simulink model "Cw3"  (R2016b)
settings: Solver=VariableStepDiscrete  StartTime=0.0  StopTime=160e-6  RelTol=1e-3
libraries: commseqgen3 x3, dspsrcs4 x2, simulink x1, commfilt2 x1, commutil2 x1
settings Model: Creator=Krzysztof  LastModifiedBy=Krzysztof

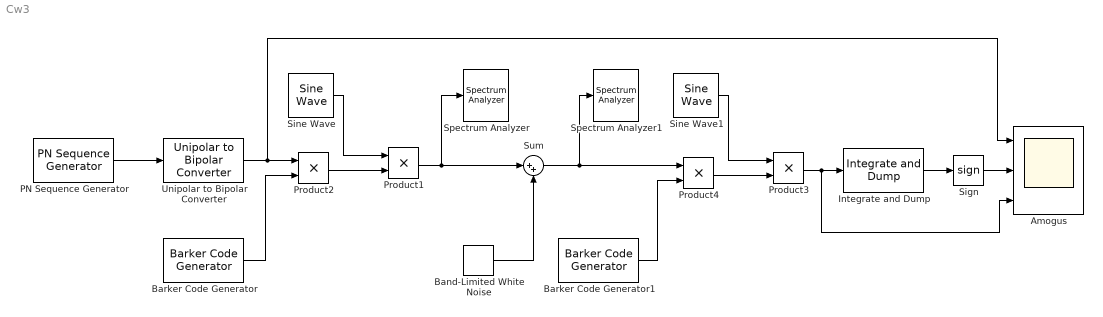
== system Cw3 ==
  "Amogus " : Scope  NumInputPorts=3
  Band-Limited White Noise : simulink/Sources/Band-Limited White Noise  Cov=[1e-11]  Ts=0.1e-9  seed=[23341]
  Barker Code Generator : commseqgen3/Barker Code Generator  Length=7  LengthSimulink=11  SampleTime=1/11e6  SamplesPerFrame=1  OutputDataType=double  SimulateUsing=Code generation
  Barker Code Generator1 : commseqgen3/Barker Code Generator  Length=7  LengthSimulink=7  SampleTime=1/11e6  SamplesPerFrame=1  OutputDataType=double  SimulateUsing=Code generation
  Integrate and Dump : commfilt2/Integrate and Dump  obssamples=10000  offsetsamples=0  nodump=off  roundingMode=Floor  overflowMode=off  outputDataTypeStr=Inherit: Same as accumulator  outputLastDataTypeStr=Inherit: Same as accumulator
  PN Sequence Generator : commseqgen3/PN Sequence Generator  poly='z^6 + z + 1'  ini_sta=[0 0 0 0 0 1]  outBitMaskSource=Dialog parameter  shift=0  outVarSiz=off  maxOutSizeMode=Dialog parameter  maxOutSize=[10 1]  Ts=1/1e6  sampPerFrame=1  reset=off  bitPackedOutputs=off  outDataType=double  numPackedBits=8  bitPackDataSigned=off  bitPackedOutDType=double
  Product1 : Product  SampleTime=0.1e-9
  Product2 : Product  SampleTime=1/11e6
  Product3 : Product  SampleTime=0.1e-9
  Product4 : Product  SampleTime=0.1e-9
  Sign : Signum
  Sine Wave : dspsrcs4/Sine Wave  Amplitude=1  Frequency=2442e6  Phase=0  SampleMode=Discrete  OutComplex=Real  CompMethod=Trigonometric fcn  TableSize=Speed  SampleTime=0.1e-9  SamplesPerFrame=1  ResetState=Restart at time zero  OutputFrames=off  dataType=double  wordLen=16  udDataType=sfix(16)  fracBitsMode=Best precision  numFracBits=15  OutDataTypeStr=double  LastOutDataTypeStr=double
  Sine Wave1 : dspsrcs4/Sine Wave  Amplitude=1  Frequency=2442e6  Phase=0  SampleMode=Discrete  OutComplex=Real  CompMethod=Trigonometric fcn  TableSize=Speed  SampleTime=0.1e-9  SamplesPerFrame=1  ResetState=Restart at time zero  OutputFrames=off  dataType=double  wordLen=16  udDataType=sfix(16)  fracBitsMode=Best precision  numFracBits=15  OutDataTypeStr=double  LastOutDataTypeStr=double
  Spectrum Analyzer : SpectrumAnalyzer
  Spectrum Analyzer1 : SpectrumAnalyzer
  Sum : Sum  Inputs=|++  SampleTime=0.1e-9
  Unipolar to Bipolar Converter : commutil2/Unipolar to Bipolar Converter  M=2  polarity=Positive  dataType=Inherit via internal rule
  wires:
  PN Sequence Generator/1 -> Unipolar to Bipolar Converter/1
  Sine Wave/1 -> Product1/1
  Product1/1 -> Sum/1, Spectrum Analyzer/1
  Barker Code Generator/1 -> Product2/2
  Product2/1 -> Product1/2
  Sine Wave1/1 -> Product3/1
  Barker Code Generator1/1 -> Product4/2
  Sum/1 -> Spectrum Analyzer1/1, Product4/1
  Product4/1 -> Product3/2
  Product3/1 -> "Amogus "/3, Integrate and Dump/1
  Integrate and Dump/1 -> Sign/1
  Unipolar to Bipolar Converter/1 -> "Amogus "/1, Product2/1
  Band-Limited White Noise/1 -> Sum/2
  Sign/1 -> "Amogus "/2
